simulink model "l8Etalon"  (R2016a)
settings: Solver=VariableStepAuto  StartTime=0.0  StopTime=10.0  RelTol=1e-3
settings Model: Creator=Student  LastModifiedBy=Student

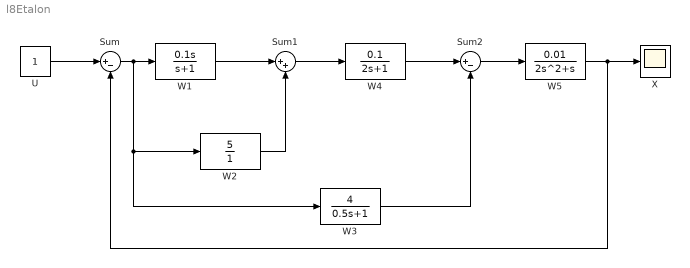
== system l8Etalon ==
  Sum : Sum  Inputs=|+-
  Sum1 : Sum  Inputs=|++
  Sum2 : Sum  Inputs=|+-
  "U " : Constant
  "W1 " : TransferFcn  Numerator=[0.1 0]  Denominator=[1 1]
  "W2 " : TransferFcn  Numerator=5  Denominator=[1]
  "W3 " : TransferFcn  Numerator=[4]  Denominator=[0.5 1]
  "W4 " : TransferFcn  Numerator=[0.1]  Denominator=[2 1]
  "W5 " : TransferFcn  Numerator=[0.01]  Denominator=[2 1 0]
  "X " : Scope
  wires:
  "U "/1 -> Sum/1
  Sum/1 -> "W3 "/1, "W2 "/1, "W1 "/1
  "W1 "/1 -> Sum1/1
  Sum1/1 -> "W4 "/1
  "W4 "/1 -> Sum2/1
  Sum2/1 -> "W5 "/1
  "W5 "/1 -> Sum/2, "X "/1
  "W2 "/1 -> Sum1/2
  "W3 "/1 -> Sum2/2
